simulink model "NXT_Motor"  (R2018b)
settings: Solver=FixedStepDiscrete  StartTime=0.0  StopTime=10.0  FixedStep=Step_Size  RelTol=1e-3
values from neighbouring files (symbols this model uses):
  Encoder_Counts_Per_Degree = Simulink.Parameter    [init.m]    (also in init_shared_parameters.m)
  Steering_Offset = Simulink.Parameter    [init.m]    (also in init_NXT_Motor.m; init_Steering_Controller.m; init_Steering_Subsystem.m = 45)
  Step_Size = 0.01    [init.m]    (also in init_shared_parameters.m)
  To_The_Left = Simulink.Parameter    [init.m]    (also in init_shared_parameters.m)
settings Model: Creator=tony  LastModifiedBy=tony
settings OptimizationCC: BlockReduction=off
settings DebuggingCC: ConsistencyChecking=error  SignalInfNanChecking=error  SignalRangeChecking=error  AlgebraicLoopMsg=error  SigSpecEnsureSampleTimeMsg=error  IntegerOverflowMsg=error  ParameterUnderflowMsg=error  ParameterPrecisionLossMsg=error  ParameterTunabilityLossMsg=error  SFcnCompatibilityMsg=error  BusObjectLabelMismatch=error  RootOutportRequireBusObject=error  AllowSymbolicDim=off  ModelReferenceVersionMismatchMessage=error  ModelReferenceIOMismatchMessage=error  UnknownTsInhSupMsg=error  StrictBusMsg=ErrorOnBusTreatedAsVector  BusNameAdapt=ErrorWithoutRepair  NonBusSignalsTreatedAsBus=error  SFInvalidInputDataAccessInChartInitDiag=error  SFTransitionOutsideNaturalParentDiag=error  SFUnreachableExecutionPathDiag=error  SFExecutionAtInitializationDiag=error  SFMachineParentedDataDiag=error  IntegerSaturationMsg=error  AllowAutomaticUnitConversions=off
settings SFSimCC: SimUseLocalCustomCode=off  SimParseCustomCode=off

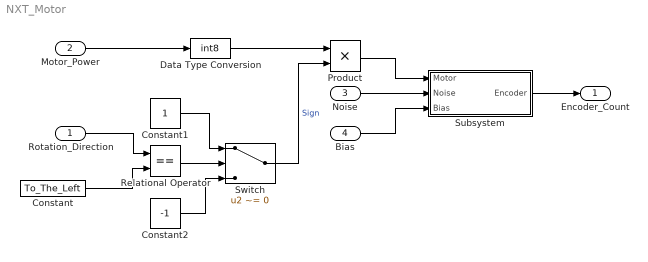
== system NXT_Motor ==
  Rotation_Direction : Inport
  Motor_Power : Inport  Port=2  OutDataTypeStr=Power_Level
  Noise : Inport  Port=3
  Bias : Inport  Port=4
  Constant : Constant  Value=To_The_Left
  Constant1 : Constant  OutDataTypeStr=int8
  Constant2 : Constant  Value=-1  OutDataTypeStr=int8
  Data Type Conversion : DataTypeConversion  OutDataTypeStr=int8  RndMeth=Zero
  Product : Product  RndMeth=Zero  InputSameDT=on  OutDataTypeStr=Inherit: Same as first input
  Relational Operator : RelationalOperator  Operator===  OutDataTypeStr=boolean  RndMeth=Simplest
  Subsystem : Subsystem
  Switch : Switch  Criteria=u2 ~= 0  Threshold=To_The_Left
  Encoder_Count : Outport
  wires:
  Subsystem/1(Encoder) -> Encoder_Count/1
  Relational Operator/1 -> Switch/2
  Rotation_Direction/1 -> Relational Operator/1
  Constant/1 -> Relational Operator/2
  Constant1/1 -> Switch/1
  Constant2/1 -> Switch/3
  Switch/1 -> Product/2  "Sign"
  Product/1 -> Subsystem/1(Motor)
  Motor_Power/1 -> Data Type Conversion/1
  Bias/1 -> Subsystem/3(Bias)
  Noise/1 -> Subsystem/2(Noise)
  Data Type Conversion/1 -> Product/1

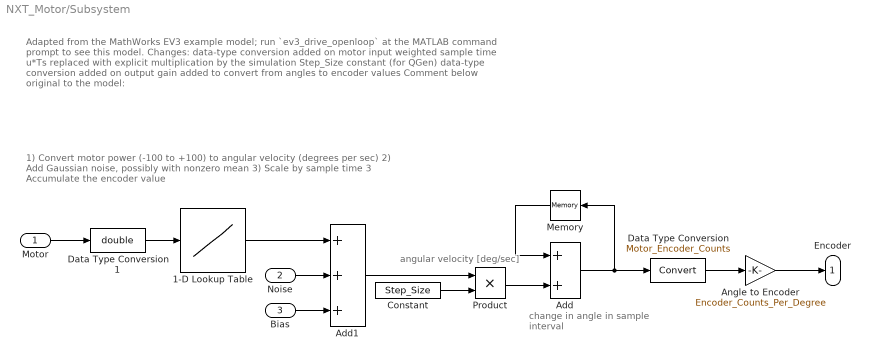
== system NXT_Motor/Subsystem ==
  note: Adapted from the MathWorks EV3 example model; run `ev3_drive_openloop` at the MATLAB command prompt to see this model.
      | Changes:
      | data-type conversion added on motor input
      | weighted sample time u*Ts replaced with explicit multiplication by the simulation Step_Size constant (for QGen)
      | data-type conversion added on output
      | gain added to convert from angles to encoder values
      |
      | Comment below original to the model:
  note: change in angle
      | in sample interval
  note: angular velocity
      |  [deg/sec]
  note: 1) Convert motor power (-100 to +100) to angular velocity (degrees per sec)
      | 2) Add Gaussian noise, possibly with nonzero mean
      | 3) Scale by sample time
      | 3 Accumulate the encoder value
  Motor : Inport
  Noise : Inport  Port=2
  Bias : Inport  Port=3
  1-D Lookup Table : Lookup_n-D  NumberOfTableDimensions=1  BreakpointsForDimension1=[-100 0 100]  Table=[-360 0 360]  ExtrapMethod=Clip  UseLastTableValue=on  RndMeth=Simplest  InputSameDT=on
  Add : Sum  AccumDataTypeStr=double  OutDataTypeStr=double
  Add1 : Sum  Inputs=+++  OutDataTypeStr=double
  Angle to Encoder : Gain  Gain=Encoder_Counts_Per_Degree  RndMeth=Zero  OutDataTypeStr=Inherit: Same as input
  Constant : Constant  Value=Step_Size
  Data Type Conversion : DataTypeConversion  OutDataTypeStr=Motor_Encoder_Counts  RndMeth=Zero
  Data Type Conversion1 : DataTypeConversion  OutDataTypeStr=double
  Memory : Memory  InitialCondition=Steering_Offset  InheritSampleTime=on  LinearizeAsDelay=on
  Product : Product  InputSameDT=on  OutDataTypeStr=Inherit: Same as first input
  Encoder : Outport
  wires:
  Noise/1 -> Add1/2
  1-D Lookup Table/1 -> Add1/1
  Add1/1 -> Product/1
  Memory/1 -> Add/1
  Motor/1 -> Data Type Conversion1/1
  Data Type Conversion/1 -> Angle to Encoder/1
  Bias/1 -> Add1/3
  Add/1 -> Data Type Conversion/1, Memory/1
  Product/1 -> Add/2
  Angle to Encoder/1 -> Encoder/1
  Constant/1 -> Product/2
  Data Type Conversion1/1 -> 1-D Lookup Table/1
